simulink model "magnetic"  (R2020b)
settings: Solver=VariableStepAuto  StartTime=0.0  StopTime=10.0  RelTol=1e-3
undefined symbols (not defined in the file): Cd, coe, day, E_prev, hours, IAU, J2, magnitude, mass, minutes, month, mu_earth, mu_moon, mu_sun, RE, S_norm, seconds, t0, v0, w_earth, WMM2020, year
libraries: vrlib x1, aerolibtransform2 x1, aerolibgravity2 x1
settings Model: Creator=khang  LastModifiedBy=khang

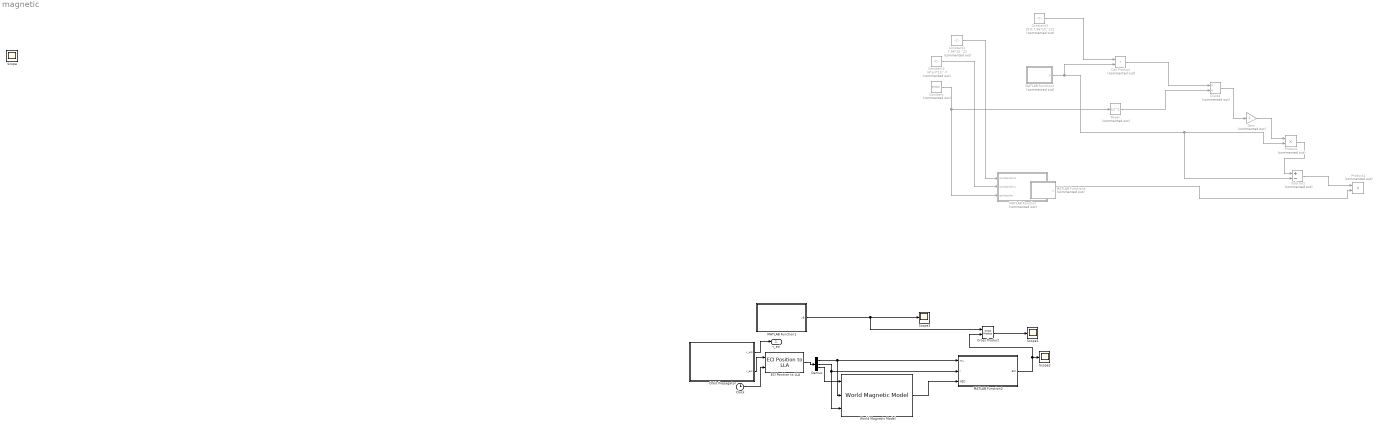
== system magnetic ==
  Clock : Clock
  Constant : Constant  Commented=on  Value=500000
  Constant1 : Constant  Commented=on  Value=7.96*10^22
  Constant2 : Constant  Commented=on  Value=(4*pi)*10^-7
  Constant3 : Constant  Commented=on  Value=[0;0;7.96*10^22]
  Cross Product : vrlib/Utilities/Cross Product
  Demux : Demux  Outputs=3
  Divide : Product  Commented=on  Inputs=*/
  Dot Product : DotProduct  Commented=on  InputSameDT=on  OutDataTypeStr=Inherit: Inherit via internal rule
  ECI Position to LLA : aerolibtransform2/ECI Position to LLA  red=IAU-2000/2006  year=2018  month=July  day=1  hour=0  min=0  sec=0  deltaT=Sec  errorflag=Error  extraparamflag=off  eunits=Metric (MKS)  earthmodel=WGS84  flat=1/298.257223563  eqradius=6378137
      settings: AttributesFormatString=%<red>  SourceProductBaseCode=AE
  Gain : Gain  Commented=on  Gain=3
  MATLAB Function : MATLAB Function  Commented=on  TreatAsAtomicUnit=on
  MATLAB Function1 : MATLAB Function  TreatAsAtomicUnit=on
  MATLAB Function2 : MATLAB Function  Commented=on  TreatAsAtomicUnit=on
  MATLAB Function3 : MATLAB Function  TreatAsAtomicUnit=on
  MATLAB Function4 : MATLAB Function  Commented=on  TreatAsAtomicUnit=on
  Orbit Propagator : Subsystem
  Power : Math  Commented=on  Operator=magnitude^2  SaturateOnIntegerOverflow=on
  Product : Product  Commented=on
  Product1 : Product  Commented=on
  Scope{,1..3} (4 alike) : Scope
  Subtract : Sum  Commented=on  Inputs=+-
  World Magnetic Model : aerolibgravity2/World Magnetic Model  model=WMM2020 (2020-2025)  customFile='WMM2020.COF'  units=Metric (MKS)  time_in=off  month=January  day=1  year=2021  action=None  h_out=off  dec_out=off  inc_out=off  ti_out=off
      settings: SourceProductBaseCode=AE
  v_eci : Outport  VectorParamsAs1DForOutWhenUnconnected=off
  wires:
  Cross Product/1 -> Scope1/1
  Constant1/1 -> MATLAB Function/1(constandmd)
  Constant2/1 -> MATLAB Function/2(constandmu)
  MATLAB Function1/1(vB) -> Cross Product/1, Scope3/1
  Constant/1 -> MATLAB Function/3(earthpolar), Power/1
  Constant3/1 -> Dot Product/1
  MATLAB Function2/1(y) -> Subtract/2, Product/2, Dot Product/2
  Dot Product/1 -> Divide/1
  Power/1 -> Divide/2
  Divide/1 -> Gain/1
  Gain/1 -> Product/1
  Product/1 -> Subtract/1
  MATLAB Function/1(vB) -> Product1/2
  Subtract/1 -> Product1/1
  ECI Position to LLA/1 -> Demux/1
  Demux/1 -> World Magnetic Model/2, MATLAB Function3/1(mu)
  Demux/2 -> World Magnetic Model/3, MATLAB Function3/2(l)
  Demux/3 -> World Magnetic Model/1
  Orbit Propagator/2(r_eci) -> ECI Position to LLA/1
  Clock/1 -> ECI Position to LLA/2
  Orbit Propagator/1(v_eci) -> v_eci/1
  World Magnetic Model/1 -> MATLAB Function3/3(NED)
  MATLAB Function3/1(ECI) -> Scope2/1, Cross Product/2

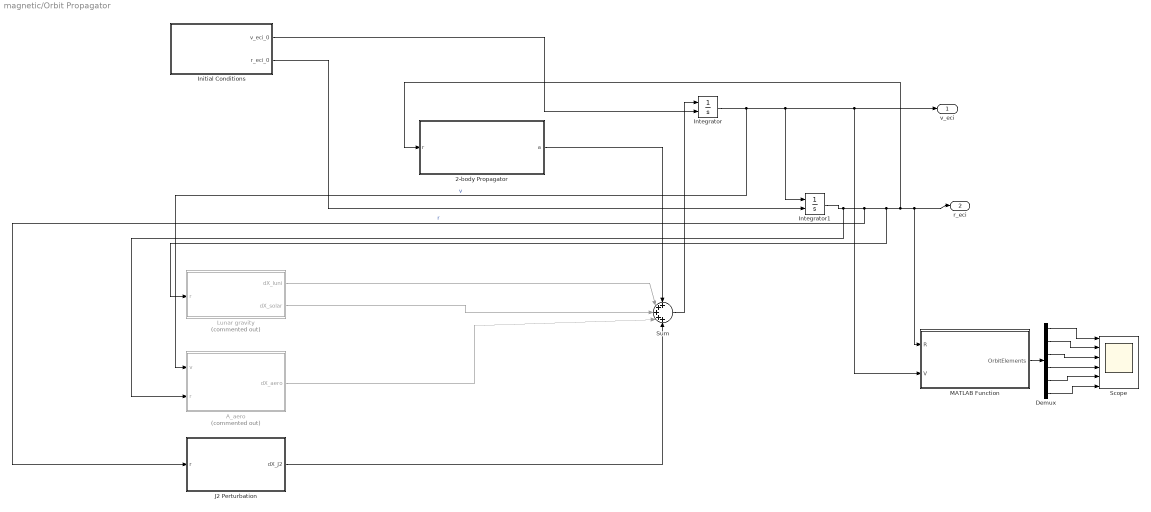
== system magnetic/Orbit Propagator ==
  2-body Propagator : Subsystem
  A_aero : Subsystem  Commented=on
  Demux : Demux  Outputs=6
  Initial Conditions : Subsystem
  Integrator : Integrator  InitialConditionSource=external  InitialCondition=v0
  Integrator1 : Integrator  InitialConditionSource=external  InitialCondition=v0
  "J2 Perturbation " : Subsystem
  Lunar gravity : Subsystem  Commented=on
  MATLAB Function : MATLAB Function  TreatAsAtomicUnit=on
  Scope : Scope  NumInputPorts=6
  Sum : Sum  Inputs=+++++
  v_eci : Outport  VectorParamsAs1DForOutWhenUnconnected=off
  r_eci : Outport  Port=2  VectorParamsAs1DForOutWhenUnconnected=off
  wires:
  Integrator1/1 -> A_aero/2(r), "J2 Perturbation "/1(r), Lunar gravity/1(r), 2-body Propagator/1(r), MATLAB Function/1(R), r_eci/1  "r"
  Integrator/1 -> A_aero/1(v), Integrator1/1, MATLAB Function/2(V), v_eci/1  "v"
  Sum/1 -> Integrator/1
  Initial Conditions/1(v_eci_0) -> Integrator/2
  Initial Conditions/2(r_eci_0) -> Integrator1/2
  2-body Propagator/1(a) -> Sum/1
  "J2 Perturbation "/1(dX_J2) -> Sum/5
  A_aero/1(dX_aero) -> Sum/4
  MATLAB Function/1(OrbitElements) -> Demux/1
  Demux/1 -> Scope/1
  Demux/2 -> Scope/2
  Demux/3 -> Scope/3
  Demux/4 -> Scope/4
  Demux/5 -> Scope/5
  Demux/6 -> Scope/6
  Lunar gravity/2(dX_solar) -> Sum/3
  Lunar gravity/1(dX_luni) -> Sum/2

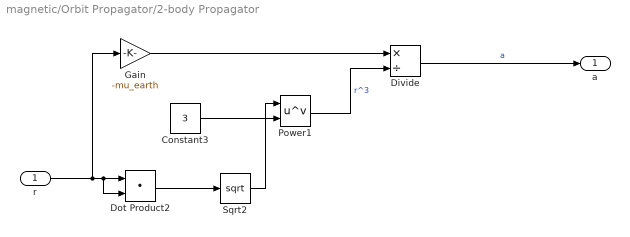
== system magnetic/Orbit Propagator/2-body Propagator ==
  r : Inport
  Constant3 : Constant  Value=3
  Divide : Product  Inputs=*/
  Dot Product2 : DotProduct  InputSameDT=on  OutDataTypeStr=Inherit: Inherit via internal rule
  Gain : Gain  Gain=-mu_earth
  Power1 : Math  Operator=pow  SignedPower=on  SaturateOnIntegerOverflow=on
  Sqrt2 : Sqrt  SaturateOnIntegerOverflow=on
  a : Outport  VectorParamsAs1DForOutWhenUnconnected=off
  wires:
  Sqrt2/1 -> Power1/1
  r/1 -> Gain/1, Dot Product2/1, Dot Product2/2
  Power1/1 -> Divide/2  "r^3"
  Gain/1 -> Divide/1
  Constant3/1 -> Power1/2
  Dot Product2/1 -> Sqrt2/1
  Divide/1 -> a/1  "a"

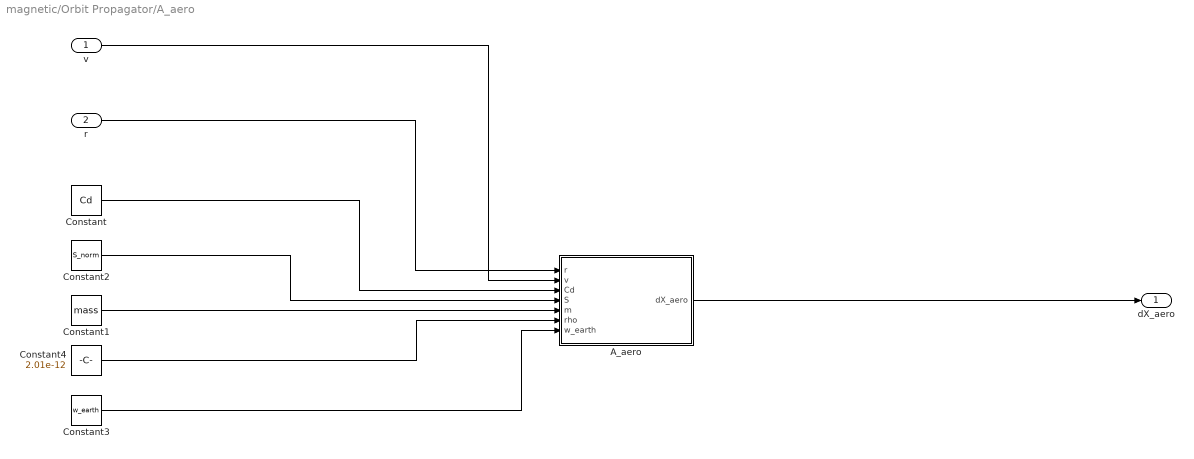
== system magnetic/Orbit Propagator/A_aero ==
  v : Inport
  r : Inport  Port=2
  A_aero : MATLAB Function  TreatAsAtomicUnit=on
  Constant : Constant  Value=Cd
  Constant1 : Constant  Value=mass
  Constant2 : Constant  Value=S_norm
  Constant3 : Constant  Value=w_earth
  Constant4 : Constant  Value=2.01e-12
  dX_aero : Outport  VectorParamsAs1DForOutWhenUnconnected=off
  wires:
  v/1 -> A_aero/2(v)
  Constant/1 -> A_aero/3(Cd)
  A_aero/1(dX_aero) -> dX_aero/1
  Constant1/1 -> A_aero/5(m)
  Constant2/1 -> A_aero/4(S)
  r/1 -> A_aero/1(r)
  Constant3/1 -> A_aero/7(w_earth)
  Constant4/1 -> A_aero/6(rho)

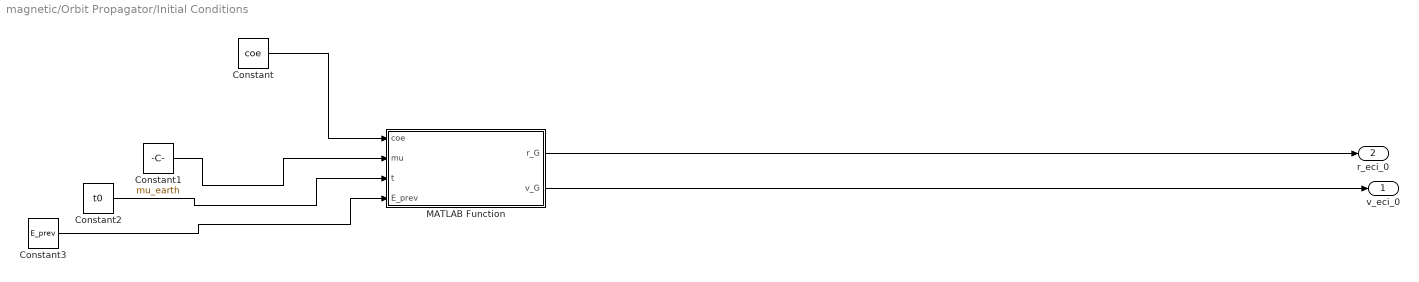
== system magnetic/Orbit Propagator/Initial Conditions ==
  Constant : Constant  Value=coe
  Constant1 : Constant  Value=mu_earth
  Constant2 : Constant  Value=t0
  Constant3 : Constant  Value=E_prev
  MATLAB Function : MATLAB Function  TreatAsAtomicUnit=on
  v_eci_0 : Outport  VectorParamsAs1DForOutWhenUnconnected=off
  r_eci_0 : Outport  Port=2  VectorParamsAs1DForOutWhenUnconnected=off
  wires:
  Constant2/1 -> MATLAB Function/3(t)
  Constant1/1 -> MATLAB Function/2(mu)
  MATLAB Function/2(v_G) -> v_eci_0/1
  Constant3/1 -> MATLAB Function/4(E_prev)
  MATLAB Function/1(r_G) -> r_eci_0/1
  Constant/1 -> MATLAB Function/1(coe)

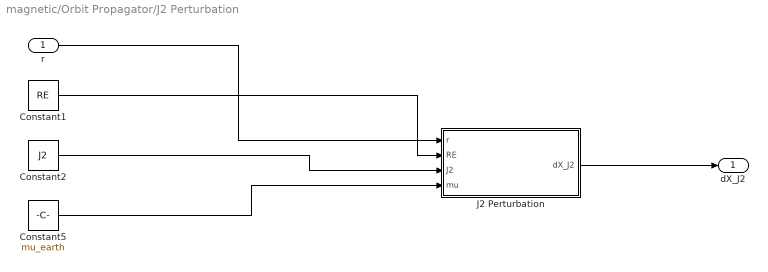
== system magnetic/Orbit Propagator/J2 Perturbation  ==
  r : Inport
  Constant1 : Constant  Value=RE
  Constant2 : Constant  Value=J2
  Constant5 : Constant  Value=mu_earth
  J2 Perturbation : MATLAB Function  TreatAsAtomicUnit=on
  dX_J2 : Outport  VectorParamsAs1DForOutWhenUnconnected=off
  wires:
  Constant5/1 -> J2 Perturbation/4(mu)
  J2 Perturbation/1(dX_J2) -> dX_J2/1
  r/1 -> J2 Perturbation/1(r)
  Constant2/1 -> J2 Perturbation/3(J2)
  Constant1/1 -> J2 Perturbation/2(RE)

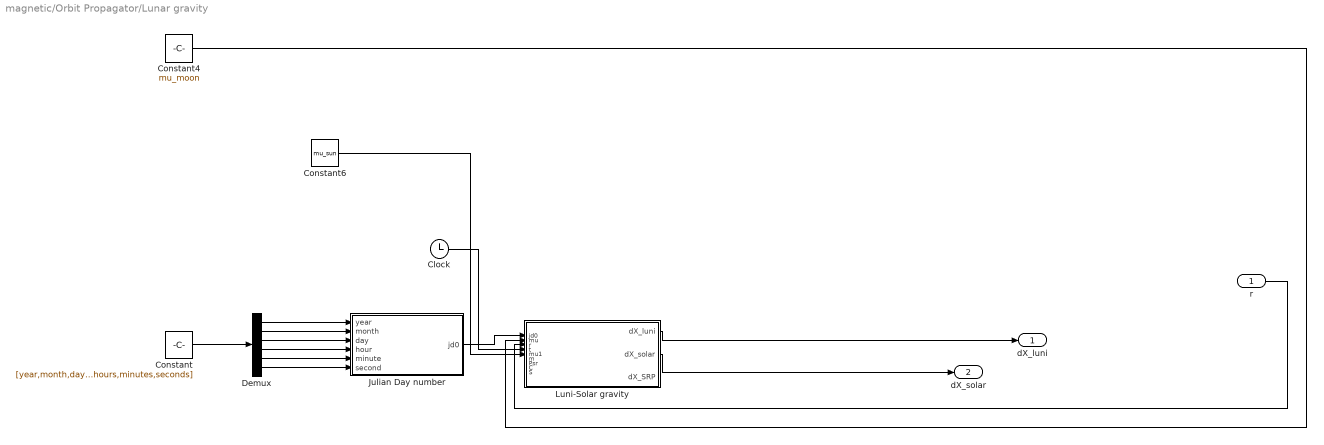
== system magnetic/Orbit Propagator/Lunar gravity ==
  r : Inport
  Clock : Clock
  Constant : Constant  Value=[year,month,day,hours,minutes,seconds]
  Constant4 : Constant  Value=mu_moon
  Constant6 : Constant  Value=mu_sun
  Demux : Demux  Outputs=6
  Julian Day number : MATLAB Function  TreatAsAtomicUnit=on
  Luni-Solar gravity : MATLAB Function  TreatAsAtomicUnit=on
  dX_luni : Outport  VectorParamsAs1DForOutWhenUnconnected=off
  dX_solar : Outport  Port=2  VectorParamsAs1DForOutWhenUnconnected=off
  wires:
  Demux/6 -> Julian Day number/6(second)
  r/1 -> Luni-Solar gravity/3(r)
  Demux/4 -> Julian Day number/4(hour)
  Constant4/1 -> Luni-Solar gravity/2(mu)
  Demux/3 -> Julian Day number/3(day)
  Demux/1 -> Julian Day number/1(year)
  Demux/5 -> Julian Day number/5(minute)
  Julian Day number/1(jd0) -> Luni-Solar gravity/1(jd0)
  Demux/2 -> Julian Day number/2(month)
  Luni-Solar gravity/1(dX_luni) -> dX_luni/1
  Constant/1 -> Demux/1
  Clock/1 -> Luni-Solar gravity/4(t)
  Luni-Solar gravity/2(dX_solar) -> dX_solar/1
  Constant6/1 -> Luni-Solar gravity/5(mu1)

== matlab function magnetic/Orbit Propagator/MATLAB Function ==
  data: R input; OrbitElements output; V input
function OrbitElements = StateVectorToOrbitElements(R,V)
%{
INPUTS:
R: Radius Vector in ECI [km]
V: Velocity Vector in ECI [km/s]

OUTPUTS:
Struct called "OrbitElements" with the format:
    'a'     Semimajor Axis [m]
    'e'     Eccentricity Magnitude
    'i'     Inclination [deg]
    'w'     Argument of Periapse [deg]
    'RAAN'  Right Ascension of the Ascending Node [deg]
    'v'     True Anomaly [deg]
    'Alt'   Altitudes of Apogee and Perigee Respectively [km]
    'FPA'	Flight Path Angle [deg]
    'OE'    Orbit Energy [MJ/kg]
%}
%% Universal Variables
r_earth = 6378137; %m
u_earth = 3.986e+14; %m^3/s^2

%Inertial Axes
I = [1; 0; 0];
J = [0; 1; 0];
K = [0; 0; 1];

%% Determine Angular Momentum
H = cross(R,V); %m^2/s

%Orbit Energy
OE = norm(V)^2/2 - u_earth/norm(R); %m^2/s^2/kg => MJ/kg

%% Determination of Eccentricity
%Eccentricity Vector
e_vector = cross(V,H)/u_earth-R/norm(R);

%Scalor Eccentricity
e = norm(e_vector);

%% Semimajor Axis 
a = -u_earth/(norm(V)^2-(2*u_earth)/norm(R)); %km

%% Determine Inclination
i = acos(dot(K,H)/(norm(K)*norm(H))); %rad

%% Determine the Right Ascension of the Ascending Node
%Node Line Vector
N = cross(K,H);

%RAAN
if N(2) < 0
    RAAN = 2*pi - acos(dot(I,N)/(norm(I)*norm(N)));
else
    RAAN = acos(dot(I,N)/(norm(I)*norm(N)));
end

%% Determine The Argument of Periapse
if e_vector(3) < 0
    w = 2*pi - acos(dot(N,e_vector)/(norm(N)*norm(e_vector)));
else
    w = acos(dot(N,e_vector)/(norm(N)*norm(e_vector)));
end

%% Determine True Anomaly
if dot(R,V) < 0
    v = 2*pi - acos(dot(e_vector,R)/(norm(e_vector)*norm(R)));
else
    v = acos(dot(e_vector,R)/(norm(e_vector)*norm(R)));
end

%% Apogee & Perigee Altitudes
%Apogee
r_a = a*(1-e^2)/(1-e); %km
    h_a = r_a - r_earth; %km

%Perigee
r_p = a*(1-e^2)/(1+e); %km
    h_p = r_p - r_earth; %km

%% Flight Path Angle
phi_fpa = atan2(e*sin(v)/sqrt(1+2*e*cos(v)+e^2),...
               (1+e*cos(v))/sqrt(1+2*e*cos(v)+e^2));

%% Format Outputs
OrbitElements = [a;e;i*180/pi;w*180/pi;RAAN*180/pi;phi_fpa*180/pi];
%StateVectorToOrbitElements.m


end

== matlab function magnetic/MATLAB Function4 ==
  data: y output
function y = fcn()

t = 0:1:2592000; %every second for a month
a = 6920*10^3;
mu = 3.986*10^14;
t0 = 0;
e = 0.007;
i = 97.4*pi/180; %radian
w = 0.005*pi/180; %rad
big_w = 229.5*pi/180; %rad
%calculate the rectum
p = a*(1 - e^2);
T = 2*pi*(a^3/mu)^(1/2)

M = sqrt(mu/a^3)*(t - t0);

E = Kepler_Newton(e,M);


theta = 2*atan(sqrt((1+e)/(1-e))*tan(E/2));

C_3w = [
        cos(w) sin(w) 0;
        -sin(w) cos(w) 0;
        0 0 1
];
C_1i = [
        1 0 0;
        0 cos(i) sin(i);
        0 -sin(i) cos(i)
];
C_3bw = [
        cos(big_w) sin(big_w) 0;
        -sin(big_w) cos(big_w) 0;
        0 0 1
];
C_oi = C_3w*C_1i*C_3bw;
C_io = C_oi.';

r = p./(1 + e.*cos(theta));

r_t = C_io*[r.*cos(theta);r.*sin(theta);zeros(size(theta))];
v_t = C_io*(mu/p)^(1/2)*[-sin(theta);cos(theta)+e;zeros(size(theta))];

%plot3(r_t(1,:),r_t(2,:),r_t(3,:))
%plot3(v_t(1,:),v_t(2,:),v_t(3,:))


for i = 1:2592001
    y = r_t(:,i);
  
end

== matlab function magnetic/MATLAB Function3 ==
  data: mu input; ECI output; l input; NED input
function ECI  = NEDtoECI(mu, l, NED)
    
    DCM = [-sin(mu)*cos(l)  -sin(mu)*sin(l)  cos(mu) ;  -sin(l)  cos(l)  0 ; -cos(mu)*cos(l)  -cos(mu)*sin(l)  -sin(mu)];
    dcmtran = DCM.';
    ned =NED.'
    disp(NED);
    ECEF = ned*dcmtran;
    utc = [2019 1 4 12 0 0];
    %ecef = ECEF.'
    DCM2 = [ cos(mu) sin(mu) 0; -sin(mu) cos(mu) 0; 0 0 1];
    dcmtran2 = DCM.';
    eci = ECEF*dcmtran2;
    ECI = eci.'
    %ECI = ecef2eci(utc,ECEF);
 
end

== matlab function magnetic/MATLAB Function1 ==
  data: vB output
function vB  = magneticresidual()
 entryone = (5+5)*rand(1);
 entrytwo = 10*rand(1);
 entrythree = 10*rand(1);
    
%lastvec = sqrt(0.002^2-entryone^2-entrytwo^2);

v = [ entryone entrytwo entrythree];
vnor = norm(v);
vb = 0.0001*[(entryone/norm(v)) (entrytwo/norm(v)) (entrythree/norm(v))];
vB = vb.'
end

== matlab function magnetic/MATLAB Function ==
  data: constandmd input; vB output; constandmu input; earthpolar input
function vB  = fludensity(constandmd,constandmu,earthpolar)

vB = (constandmu*constandmd)/4*pi*earthpolar

== matlab function magnetic/MATLAB Function2 ==
  data: y output
function y = fcn()

t = 0:1:2592000; %every second for a month
a = 6920*10^3;
mu = 3.986*10^14;
t0 = 0;
e = 0.007;
i = 97.4*pi/180; %radian
w = 0.005*pi/180; %rad
big_w = 229.5*pi/180; %rad
%calculate the rectum
p = a*(1 - e^2);
T = 2*pi*(a^3/mu)^(1/2)

M = sqrt(mu/a^3)*(t - t0);

E = Kepler_Newton(e,M);


theta = 2*atan(sqrt((1+e)/(1-e))*tan(E/2));

C_3w = [
        cos(w) sin(w) 0;
        -sin(w) cos(w) 0;
        0 0 1
];
C_1i = [
        1 0 0;
        0 cos(i) sin(i);
        0 -sin(i) cos(i)
];
C_3bw = [
        cos(big_w) sin(big_w) 0;
        -sin(big_w) cos(big_w) 0;
        0 0 1
];
C_oi = C_3w*C_1i*C_3bw;
C_io = C_oi.';

r = p./(1 + e.*cos(theta));

r_t = C_io*[r.*cos(theta);r.*sin(theta);zeros(size(theta))];
v_t = C_io*(mu/p)^(1/2)*[-sin(theta);cos(theta)+e;zeros(size(theta))];

%plot3(r_t(1,:),r_t(2,:),r_t(3,:))
%plot3(v_t(1,:),v_t(2,:),v_t(3,:))


for i = 1:2592001
    y = r_t(:,i);
  
end

== matlab function magnetic/Orbit Propagator/A_aero/A_aero ==
  data: r input; dX_aero output; v input; Cd input; S input; m input; rho input; w_earth input
function dX_aero = Aero(r,v,Cd,S,m,rho,w_earth)
sg = (Cd*S/2*m);
va = v - cross(w_earth,r);
v_a = norm(va);

dX_aero = sg*rho*(v_a^2)*(va/v_a);

end

== matlab function magnetic/Orbit Propagator/Initial Conditions/MATLAB Function ==
  data: coe input; r_G output; mu input; t input; E_prev input; v_G output
function [r_G,v_G] = OrbMech(coe,mu, t, E_prev)
%ORBMECH models the orbital mechanics of the spacecraft
%   Assuming an ideal, non-perturbed orbit, the position of
%   the spacecraft (in the inertial frame) is determined, using the ISS
%   orbital elements

a = coe(1);e=coe(2);i=coe(3);raan=coe(4);w = coe(5);t0=coe(6);

% Solve for Eccentric Anomaly (E)
E_fun = @(E) E-e*sin(E) - sqrt(mu/a^3) * (t-t0);
E = fzero(E_fun,E_prev);

% Solve for True Anomaly (theta)
theta = 2*atan2(sqrt(1+e)*sin(E/2),sqrt(1-e)*cos(E/2));

% Compute SC position vector in the ECI frame (r_G)
r = a*(1 - e*cos(E));
ci=cos(i); co=cos(raan); cw=cos(w);si=sin(i); so=sin(raan); sw=sin(w);
C_PG = [cw*co-sw*ci*so, cw*so+sw*ci*co, sw*si;
        -sw*co-cw*ci*so, -sw*so+cw*ci*co, cw*si;
        si*so, -si*co, ci];
C_GP = C_PG';

% Compute SC position & velocity vector in the ECI frame
vel=sqrt(mu/a*(1-e^2))*[-sin(theta);e+cos(theta);0]; % Velocity vector of s/c in perifocal plane
r_G = C_GP * [r*cos(theta); r*sin(theta); 0];
v_G= C_GP* vel;

end

== matlab function magnetic/Orbit Propagator/J2 Perturbation /J2 Perturbation ==
  data: r input; dX_J2 output; RE input; J2 input; mu input
function dX_J2 = J2(r,RE,J2,mu)
rpp = norm(r);
xx = r(1); yy = r(2); zz = r(3);
fac = 3/2*J2*(mu/rpp^2)*(RE/rpp)^2;
dX_J2 = -fac*[(1 - 5*(zz/rpp)^2)*(xx/rpp) ...
(1 - 5*(zz/rpp)^2)*(yy/rpp) ...
(3 - 5*(zz/rpp)^2)*(zz/rpp)];
end

== matlab function magnetic/Orbit Propagator/Lunar gravity/Julian Day number ==
  data: year input; jd0 output; month input; day input; hour input; minute input; second input
function jd0 = JDnumber(year,month,day,hour,minute,second)
% Calculates the JD number for a given year,month and day

j0 = 367*year - fix(7*(year + fix((month + 9)/12))/4) + fix(275*month/9) + day + 1721013.5; 

ut = hour + minute/60 + second/3600; % UTC time in hour format

jd0 = j0 + ut/24; % JD number calculation


end

== matlab function magnetic/Orbit Propagator/Lunar gravity/Luni-Solar gravity ==
  data: jd0 input; dX_luni output; mu input; r input; t input; mu1 input; dX_solar output; m input; Psr input; C input; S input; dX_SRP output
function [dX_luni,dX_solar,dX_SRP] = LuniSolar(jd0,mu,r,t,mu1,m,Psr,C,S)
% Moon gravity contribution
jd_new = jd0 + t/86400;
R_moon = Lunargravity(jd_new);
R_ms = R_moon - r;
r_ms = norm(R_ms);
r_moon = norm(R_moon);

% Sun gravity contribution
[R_sun,u_sun] = Solargravity(jd_new);
lswitch = los(r,R_sun);
r_sun = norm(R_sun);
R_ss = R_sun - r;
r_ss = norm(R_ss);
q = dot(r,(2*R_sun - r))/r_sun^2;
Fq = q*(q^2 - 3*q +3)/(1 + sqrt(1-q));
%% SRP terms
psr = (lswitch*Psr*C*S)/m;

dX_luni = mu*((R_ms/r_ms^3) - (R_moon/r_moon^3));
dX_solar = (mu1/r_ss^3)*(Fq*R_sun - r);
dX_SRP = -psr*u_sun;
end
